simulink model "S_simulink_full_test"  (R2022b)
settings: Solver=VariableStepAuto  StartTime=0.0  StopTime=100  RelTol=1e-3
settings Model: Creator=user  LastModifiedBy=user

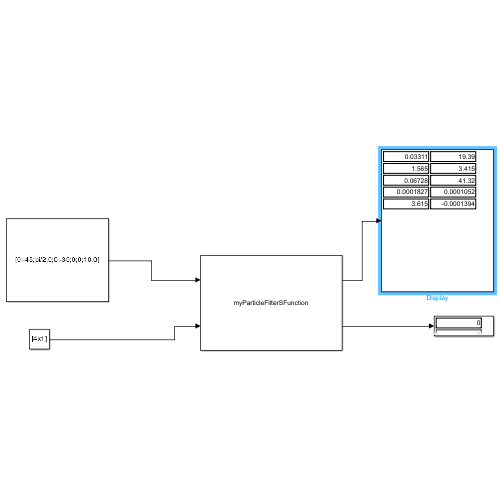
[thumbnail: Simulink's stored preview of the top-level diagram]
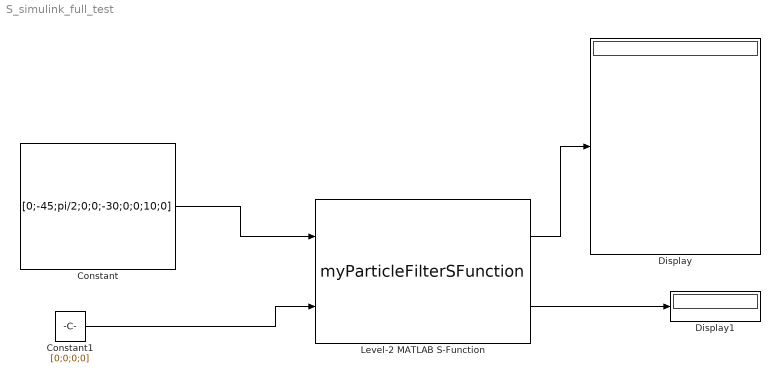
== system S_simulink_full_test ==
  Constant : Constant  Value=[0;-45;pi/2;0;0;-30;0;0;10;0]
  Constant1 : Constant  Value=[0;0;0;0]
  Display : Display
  Display1 : Display
  Level-2 MATLAB S-Function : M-S-Function  FunctionName=myParticleFilterSFunction
  wires:
  Constant/1 -> Level-2 MATLAB S-Function/1
  Constant1/1 -> Level-2 MATLAB S-Function/2
  Level-2 MATLAB S-Function/1 -> Display/1
  Level-2 MATLAB S-Function/2 -> Display1/1
